simulink library "cm_custom"  (R2018b)
settings: Solver=VariableStepAuto  StartTime=0.0  StopTime=10.0  RelTol=1e-3
undefined symbols (not defined in the file or in its folder): DiscIntNeverNeededParam
libraries: simulink x19, raspberrypilib x4, $bdroot x2, speedgoatlib_fpga x2, androidcommunicationlib x1, embdlinuxlib x1, commutil2 x1
(part 2 of 2)

== stateflow chart cm_custom/RPi I2C MPU6050 ==
  state initialization_sequence
    entry:
    imu_rdy = 0;
    state reset
      during:
      imu_err = dev_reset();
      state err = dev_reset [function]
    state parsing
    state settings
      entry:
      imu_err = init_2();
      state err = init_2 [function]
    state wakeup
      entry:
      imu_err = init_1();
      state err = init_1 [function]
    state parsing1
    state parsing2
    (default) -> reset
    settings -> reset [order 2]
    reset -> parsing : [imu_err == 0]
    wakeup -> reset [order 2]
    parsing -> wakeup : after(0.5, sec)
    wakeup -> parsing1 [order 1] : [imu_err==0]
    parsing1 -> settings : after(0.2,sec)
    settings -> parsing2 [order 1] : [imu_err==0]
  state read_atg
    during:
    state [acc,temp,gyro,err] = read_raw_atg [function]
    state badRead
    state goodRead
      entry:
      raw_acc_calibrated[0] = (double(raw_acc[0]) * PAR_SENS_ACC[0]) + PAR_OFFSET_ACC[0];
      raw_acc_calibrated[1] = (double(raw_acc[1]) * PAR_SENS_ACC[1]) + PAR_OFFSET_ACC[1];
      raw_acc_calibrated[2] = (double(raw_acc[2]) * PAR_SENS_ACC[2]) + PAR_OFFSET_ACC[2];
      raw_gyro_calibrated[0] = (double(raw_gyro[0]) * PAR_SENS_GYRO[0]) + PAR_OFFSET_GYRO[0];
      raw_gyro_calibrated[1] = (double(raw_gyro[1]) * PAR_SENS_GYRO[1]) + PAR_OFFSET_GYRO[1];
      raw_gyro_calibrated[2] = (double(raw_gyro[2]) * PAR_SENS_GYRO[2]) + PAR_OFFSET_GYRO[2];
      imu_rdy = 1;
    badRead -> (junction 151) [order 2]
    (junction 155) -> badRead [order 2] : {n_badRead++;}
    (junction 151) -> (junction 155) : {[raw_acc, raw_temp, raw_gyro, imu_err] = read_raw_atg();}
    (junction 155) -> goodRead [order 1] : [imu_err==0]{n_badRead=0;}
    goodRead -> (junction 151)
  (default) -> initialization_sequence
  parsing2 -> (junction 151) : after(1, sec)
  badRead -> initialization_sequence [order 1] : [n_badRead >= 10]{imu_rdy = 0;}
  data: err function_output; err function_output; err function_output; acc function_output; temp function_output; gyro function_output; err function_output uint8; write_buffer local uint8 size=63; read_err local boolean size=1; write_err local boolean size=1; read_buffer local uint8 size=64; raw_acc local int16 size=3; raw_gyro local int16 size=3; raw_temp local int16 size=1; raw_acc_calibrated output double size=3 =[0 0 -9.80665]; raw_gyro_calibrated output double size=3 =[0 0 0]; PAR_OFFSET_ACC parameter double size=3; PAR_OFFSET_GYRO parameter double size=3; PAR_SENS_ACC parameter double size=3; PAR_SENS_GYRO parameter double size=3; imu_rdy output uint8; imu_err local uint8; n_badRead local uint32

== matlab function cm_custom/spherical qw ==
  data: pqr input; qw output; dt input
function qw = fcn(pqr, dt)


qw = [1 0 0 0];
npqr = sqrt(pqr(1)^2 + pqr(2)^2 + pqr(3)^2);
cnxb2 = cos(npqr * dt / 2);
snxb2 = sqrt(1 - cnxb2^2);
qw(1) = cnxb2;
qw(2:4) = pqr ./ npqr * snxb2;

== matlab function cm_custom/RT Derivative (x:[-pi pi])/short side ==
  data: u input; y output
function y = fcn(u)
persistent m
if isempty(m)
    m = length(u);
end

y = u;

parfor i = 1:m
    if y(i) > pi
        y(i) = y(i) - 2*pi;
    elseif y(i) <= -pi
        y(i) = y(i) + 2*pi;
    end
end

== matlab function cm_custom/Saturated Double Integrator/MATLAB Function ==
  data: ddxo input; x0 input; dx0 input; max_x input; min_x input; max_dx input; min_dx input; Ts input; init input; x output; dx output; ddx output
function [x, dx, ddx] = outputSatDoubleInt(ddxo, x0, dx0, max_x, min_x, max_dx, min_dx, Ts, init)

persistent xo dxo 
if isempty(xo)
    xo = x0;
    dxo = dx0;
end

if init
    xo = x0;
    dxo = dx0;
end

%% native integration
x = xo + dxo * Ts + 0.5 * ddxo * Ts^2;
dx = dxo + ddxo * Ts;
ddx = ddxo;

%% zero derivatives upon limit
dx = dx .* double((x >= min_x) & (x <= max_x));
ddx = ddx .* double((x >= min_x) & (x <= max_x));

ddx = ddx .* double((dx >= min_dx) & (dx <= max_dx));

%% limit
x = x .* double((x >= min_x) & (x <= max_x)) ...
    + max_x .* double(x > max_x) ...
    + min_x .* double(x < min_x);

dx = dx .* double((dx >= min_dx) & (dx <= max_dx)) ...
    + max_dx .* double(dx > max_dx) ...
    + min_dx .* double(dx < min_dx);

%% assign old
xo = x;
dxo = dx;

== stateflow chart cm_custom/Free Fall Trigger ==
  state idle
    entry:
    freeFall = 0;
  state lowGing
  state idle1
    entry:
    freeFall = 0;
  state FREEEFALLL
    entry:
    freeFall = 1;
  (default) -> idle
  idle -> lowGing : [lowG == 1]
  lowGing -> FREEEFALLL [order 2] : after(0.05, sec)
  lowGing -> idle [order 1] : [lowG == 0]
  idle1 -> idle : after(1, sec)
  FREEEFALLL -> idle1 : after(freeFallTime, sec) [lowG == 0]
  data: lowG input boolean size=1; freeFall output boolean size=1 =0; freeFallTime input

== matlab function cm_custom/EKF/EKF ==
  data: fuse input; y input; xh input; yh input; A input; B input; C input; Qo input; R input; Po input; x output; P output
function [x, P] = EKF(fuse, y, xh, yh, A, B, C, Qo, R, Po)

persistent nx
if isempty(nx)
    nx = length(xh);
end

x = xh;
P = A * Po * A' + Qo;

if fuse
    K = P * C' * (C * P * C' + R)^-1;
    x = xh + K * (y - yh);
    G = eye(nx) - K * C;
    P = G * P * G' + K * R * K';
end

== matlab function cm_custom/SFB m2a ==
  data: pitch output; yaw output; J_dm2dpy output; the1 input; the2 input; J_dpy2dm output
function [pitch, yaw, J_dm2dpy, J_dpy2dm] = fcn(the1, the2)


r = 1;
w = 1;

thep = (the1 + the2) / 2;
thed = (the1 - the2) / 2;

M = [thep; atan(-2*r/w*sin(thed))];
pitch = M(1);
yaw = M(2);

% singularity protection
% if (abs(thed) > 30*pi/180)
%     thed = sign(thed) * 30*pi/180;
% end
dM_dthepthed = [1 0;
                0 ((-2*r*cos(thed))*w)/(w^2 + 4*r^2*sin(thed)^2)];
dthepthed_dthe1the2 = [1/2 1/2; 1/2 -1/2];

J_dm2dpy = dM_dthepthed * dthepthed_dthe1the2;

J_dpy2dm = J_dm2dpy';
